simulink model "Ex7_IC"  (R2021a)
settings: Solver=VariableStepAuto  StartTime=0.0  StopTime=10.0  RelTol=1e-3
undefined symbols (not defined in the file): fdesignblkfcn, gcbh
libraries: dspfdesign x1
settings Model: Creator=gferr  LastModifiedBy=gferr

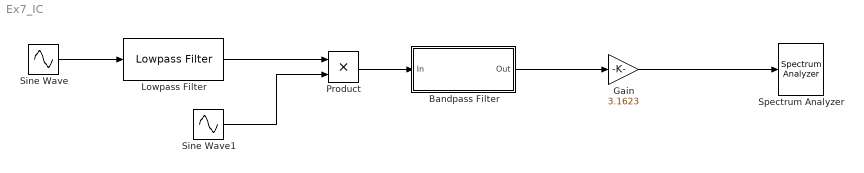
== system Ex7_IC ==
  Bandpass Filter : Subsystem  DialogController=fdesignblkfcn  InitFcn=fdesignblkfcn(gcbh, {'InitFcn'});  mask(Bandpass Filter){}
      mask help: Design a bandpass filter
      settings: CopyFcn=fdesignblkfcn(gcbh, {'CopyFcn'});
      mask Help: helpview(mapfilelocation('dsp'), 'dspbandpassfilter');
      mask Display: disp('Bandpass');
  Gain : Gain  Gain=3.1623
  Lowpass Filter : dspfdesign/Lowpass Filter  FilterType=FIR  DesignForMinimumOrder=on  FilterOrder=50  PassbandFrequency=8e3  StopbandFrequency=12e3  PassbandRipple=0.1  StopbandAttenuation=80  InheritSampleRate=off  SampleRate=44100  SimulateUsing=Interpreted execution  roundingMode=Floor  coeffsDataTypeStr=fixdt(1,16)
  Product : Product
  Sine Wave : Sin  Amplitude=0.5  Frequency=2*pi*500  SampleTime=1/44100
  Sine Wave1 : Sin  Frequency=2*pi*5000  SampleTime=1/44100
  Spectrum Analyzer : SpectrumAnalyzer
  wires:
  Sine Wave/1 -> Lowpass Filter/1
  Lowpass Filter/1 -> Product/1
  Sine Wave1/1 -> Product/2
  Product/1 -> Bandpass Filter/1(In)
  Bandpass Filter/1(Out) -> Gain/1
  Gain/1 -> Spectrum Analyzer/1

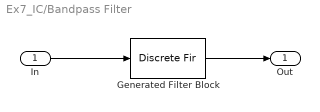
== system Ex7_IC/Bandpass Filter ==
  In : Inport
  Generated Filter Block : DiscreteFir  Tag=BlockMethodSubSystem  Coefficients=[-0.0688259615692904392 0.0570912116969295863 0.0417993046089595172 0.0303961422695806227 0.0197234046037490854 0.0095241061109775562 0.0015656059989722043 -0.00220448701905183366 -0.00128691037626906348 0.0027024125856537351 0.00668967245330745648 0.00779842088042472306 0.00497693106396991398 -0.00043642262138559435 -0.00544207760248957648 -0.00716202856571789784 -0.00456838410967588468 0.000858112838227520231 0.00595139687799145414 0.00768288246213540572 0.00495471906188731884 -0.000727487947714666803 -0.00608285478535723189 -0.00795066481523758022 -0.00516911900687324222 0.0007130322379219411 0.00627464487802291068 0.00824377183163470945 0.00539522533805542222 -0.000681911213243298234 -0.00647990927177880243 -0.00854534367501845644 -0.00564700003796811487 0.000623341402462660767 0.00661318598124289829 0.00882055975185886028 0.00583862820931205749 -0.000542411269245878761 -0.00682968619759920671 -0.00903526097825343988 -0.00606831206231513848 0.000455907849588848733 0.00696837620778019938 0.00931563860889562598 0.0062155683946489718 -0.000562858060195403414 -0.0070337598710713909 -0.00950250665653370151 -0.00642238708071405946 0.000418761202999837342 0.00711941637757688289 0.00968867277197305032 0.00662411491828814643 -0.000368662840708789492 -0.00717819396921931443 -0.00985391517359167877 -0.00675409457423065736 0.000296484297314922047 0.00722863816001276509 0.00993813537686809995 0.00686295321035839713 -0.000255136141318648073 -0.00723810546101213807 -0.0100449837488797537 -0.00697325120086811877 0.000178998130159601938 0.00728771305610552769 0.0101315835951310221 0.00707326164730153178 -0.000118434141431750099 -0.00724240071399064392 -0.0101971879880789155 -0.00714138430753517937 3.96193385966688521e-05 0.00722103115071584013 0.0102010033284814332 0.00722103115071584013 3.96193385966688521e-05 -0.00714138430753517937 -0.0101971879880789155 -0.00724240071399064392 -0.000118434141431750099 0.00707326164730153178 0.0101315835951310221 0.00728771305610552769 0.000178998130159601938 -0.00697325120086811877 -0.0100449837488797537 -0.00723810546101213807 -0.000255136141318648073 0.00686295321035839713 0.00993813537686809995 0.00722863816001276509 0.000296484297314922047 -0.00675409457423065736 -0.00985391517359167877 -0.00717819396921931443 -0.000368662840708789492 0.00662411491828814643 0.00968867277197305032 0.00711941637757688289 0.000418761202999837342 -0.00642238708071405946 -0.00950250665653370151 -0.0070337598710713909 -0.000562858060195403414 0.0062155683946489718 0.00931563860889562598 0.00696837620778019938 0.000455907849588848733 -0.00606831206231513848 -0.00903526097825343988 -0.00682968619759920671 -0.000542411269245878761 0.00583862820931205749 0.00882055975185886028 0.00661318598124289829 0.000623341402462660767 -0.00564700003796811487 -0.00854534367501845644 -0.00647990927177880243 -0.000681911213243298234 0.00539522533805542222 0.00824377183163470945 0.00627464487802291068 0.0007130322379219411 -0.00516911900687324222 -0.00795066481523758022 -0.00608285478535723189 -0.000727487947714666803 0.00495471906188731884 0.00768288246213540572 0.00595139687799145414 0.000858112838227520231 -0.00456838410967588468 -0.00716202856571789784 -0.00544207760248957648 -0.00043642262138559435 0.00497693106396991398 0.00779842088042472306 0.00668967245330745648 0.0027024125856537351 -0.00128691037626906348 -0.00220448701905183366 0.0015656059989722043 0.0095241061109775562 0.0197234046037490854 0.0303961422695806227 0.0417993046089595172 0.0570912116969295863 -0.0688259615692904392]  InputProcessing=Columns as channels (frame based)
  Out : Outport  VectorParamsAs1DForOutWhenUnconnected=off
  wires:
  In/1 -> Generated Filter Block/1
  Generated Filter Block/1 -> Out/1
